simulink model "PX4OutputMappingEvtolSimscape"  (R2026a)
settings: configuration reference "standardSILConfiguraitonParams" (kept outside this file)
undefined symbols (not defined in the file): MotorCommandHexBus
settings Model: Creator=jerem  LastModifiedBy=Edison Altamirano
settings ConfigSetRef: SourceName=standardSILConfiguraitonParams  SourceLocation=Base Workspace

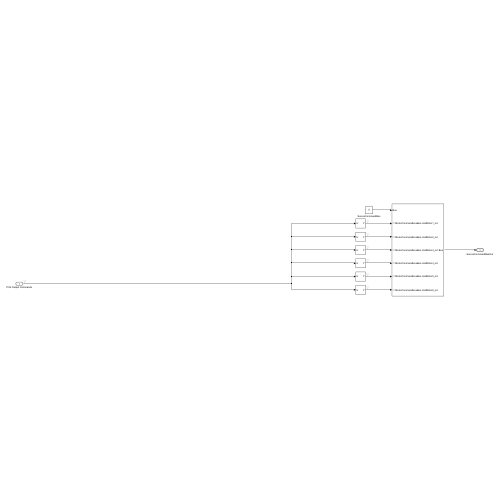
[thumbnail: Simulink's stored preview of the top-level diagram]
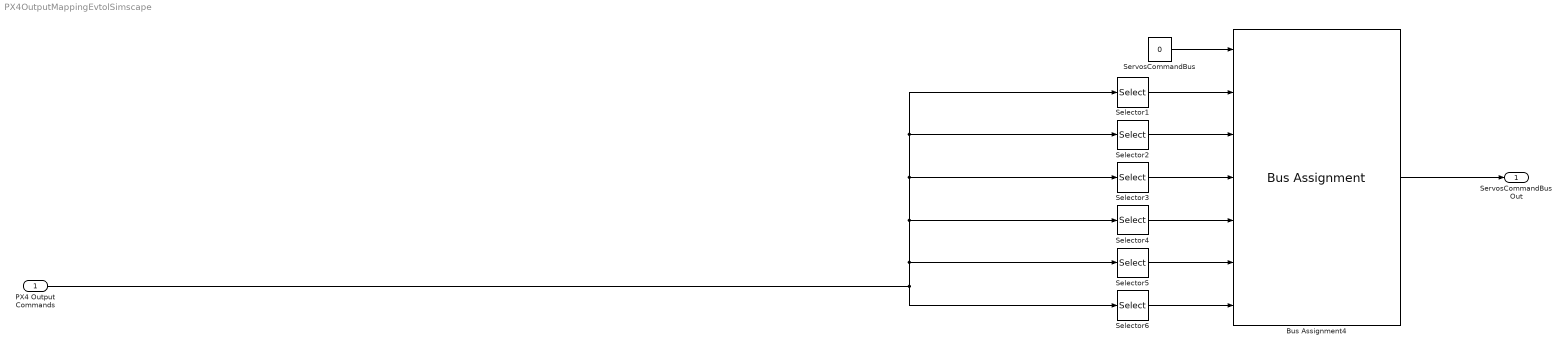
== system PX4OutputMappingEvtolSimscape ==
  PX4 Output Commands : Inport  PortDimensions=16
  Bus Assignment4 : BusAssignment  AssignedSignals=MotorCommandHexBus.cmdRotor1_nd,MotorCommandHexBus.cmdRotor2_nd,MotorCommandHexBus.cmdRotor3_nd,MotorCommandHexBus.cmdRotor4_nd,MotorCommandHexBus.cmdRotor5_nd,MotorCommandHexBus.cmdRotor6_nd
  Selector1 : Selector  InputPortWidth=16  IndexOptions=Index vector (dialog)  Indices=1  OutputSizes=1
  Selector2 : Selector  InputPortWidth=16  IndexOptions=Index vector (dialog)  Indices=2  OutputSizes=1
  Selector3 : Selector  InputPortWidth=16  IndexOptions=Index vector (dialog)  Indices=3  OutputSizes=1
  Selector4 : Selector  InputPortWidth=16  IndexOptions=Index vector (dialog)  Indices=4  OutputSizes=1
  Selector5 : Selector  InputPortWidth=16  IndexOptions=Index vector (dialog)  Indices=5  OutputSizes=1
  Selector6 : Selector  InputPortWidth=16  IndexOptions=Index vector (dialog)  Indices=6  OutputSizes=1
  ServosCommandBus : Constant  Value=0  OutDataTypeStr=Bus: ServosCommandBus
  ServosCommandBusOut : Outport  OutDataTypeStr=Bus: ServosCommandBus
  wires:
  ServosCommandBus/1 -> Bus Assignment4/1
  Bus Assignment4/1 -> ServosCommandBusOut/1
  PX4 Output Commands/1 -> Selector1/1, Selector2/1, Selector3/1, Selector4/1, Selector5/1, Selector6/1
  Selector1/1 -> Bus Assignment4/2
  Selector2/1 -> Bus Assignment4/3
  Selector3/1 -> Bus Assignment4/4
  Selector4/1 -> Bus Assignment4/5
  Selector5/1 -> Bus Assignment4/6
  Selector6/1 -> Bus Assignment4/7
